simulink model "motoraiHIL"  (R2018b)
settings: Solver=FixedStepDiscrete  StartTime=0.0  StopTime=inf  FixedStep=SAMPLE_TIME  RelTol=1e-3
InitFcn:
  | UserSettings
values from neighbouring files (symbols this model uses):
  ADC_bits = 12    [LQR_control_design.m]    (also in UserSettings.m)
  ADC_Vref = 3.3    [LQR_control_design.m]    (also in UserSettings.m)
  current_gain = 0.5    [LQR_control_design.m]    (also in UserSettings.m)
  current_offset = 1    [LQR_control_design.m]    (also in UserSettings.m)
  DATA_SAMPLING_FREQUENCY = 500    [UserSettings.m]
  ESTIMATION_SAMPLES = 50    [UserSettings.m]
  i_max = 20    [LQG_control_design.m]    (also in LQR_control_design.m; UserSettings.m)
  motorParameters = Parameters()    [UserSettings.m]
  omega_gain = 0.5    [LQR_control_design.m]    (also in UserSettings.m)
  omega_max = 20    [LQG_control_design.m]    (also in LQR_control_design.m; UserSettings.m)
  omega_offset = 1    [LQR_control_design.m]    (also in UserSettings.m)
  PPR = 1000    [LQR_control_design.m]    (also in UserSettings.m)
  SAMPLE_TIME = 5e-5    (= 5e-05)    [UserSettings.m]
  V_ACT = 12    [UserSettings.m]
  v_max = 10    [LQG_control_design.m]    (also in LQR_control_design.m; UserSettings.m)
undefined symbols (not defined in the file or in its folder): myLQR, myREF, parameter_ranges
libraries: neural x230, mbedblockslib x7, dspswit3 x2, dspbuff3 x2, powerlib_meascontrol x2, discretizing x1
(part 1 of 11)
settings Model: ExtModeTrigDuration=10  Creator=Filippo  LastModifiedBy=Filippo
settings OptimizationCC: DefaultParameterBehavior=Inlined  UseDivisionForNetSlopeComputation=on  UseFloatMulNetSlope=on  UseSpecifiedMinMax=on  InlineInvariantSignals=on  EnhancedBackFolding=on  BooleansAsBitfields=on  PassReuseOutputArgsAs=Individual arguments  StateBitsets=on  DataBitsets=on  ZeroExternalMemoryAtStartup=off  ZeroInternalMemoryAtStartup=off  NoFixptDivByZeroProtection=on  EfficientFloat2IntCast=on  LifeSpan=1  MaxStackSize=64  OptimizeBlockOrder=speed  DifferentSizesBufferReuse=on
settings DebuggingCC: SignalInfNanChecking=error  IntegerOverflowMsg=error  ParameterTunabilityLossMsg=error  AssertControl=DisableAll  SFUndirectedBroadcastEventsDiag=error
settings HardwareCC: ProdBitPerPointer=32  ProdBitPerSizeT=32  ProdBitPerPtrDiffT=32  ProdLargestAtomicInteger=Long  ProdLargestAtomicFloat=Double  ProdWordSize=32  ProdLongLongMode=on  ProdHWDeviceType=ARM Compatible->ARM Cortex
settings SFSimCC: CompileTimeRecursionLimit=0  EnableRuntimeRecursion=off  MATLABDynamicMemAlloc=off
settings RTWCC: SystemTargetFile=ert.tlc  HardwareBoard=STM32 Nucleo F411RE  TemplateMakefile=ert_default_tmf  GenerateReport=on  Toolchain=GNU Tools for ARM Embedded Processors  BuildConfiguration=Faster Runs  IncludeHyperlinkInReport=on  LaunchReport=on  GenerateTraceInfo=on  GenerateTraceReport=on  GenerateTraceReportSl=on  GenerateTraceReportSf=on  GenerateTraceReportEml=on  GenerateCodeMetricsReport=on
settings CodeAppCC: ForceParamTrailComments=on  IgnoreCustomStorageClasses=off  OperatorAnnotations=on  SimulinkDataObjDesc=on  SFDataObjDesc=on  CustomSymbolStrGlobalVar=rt$N$M  CustomSymbolStrType=$N$M  CustomSymbolStrFcn=$N$M$F  CustomSymbolStrMacro=$N$M  InsertBlockDesc=on
settings ERTTargetCC: UtilityFuncGeneration=Shared location  IncludeMdlTerminateFcn=off  CombineSignalStateStructs=on  SupportAbsoluteTime=off  SupportComplex=off  SupportNonInlinedSFcns=on  SupportVariableSizeSignals=on  ParenthesesLevel=Maximum  CastingMode=Standards  GenerateSharedConstants=off  InlinedParameterPlacement=NonHierarchical  ERTFilePackagingFormat=CompactWithDataFile  EnableSignedLeftShifts=off  EnableSignedRightShifts=off

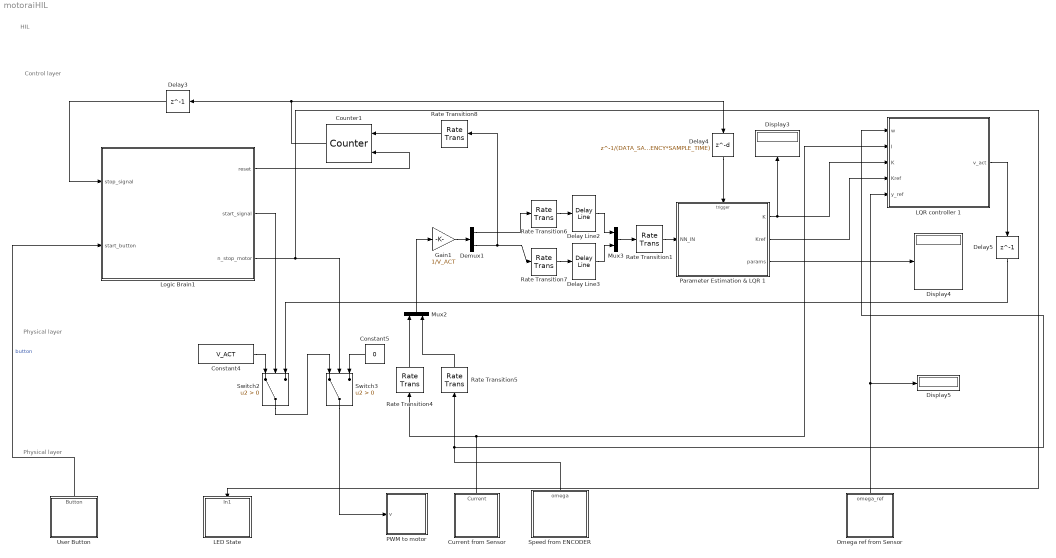
== system motoraiHIL ==
  note: Physical layer
  note: Control layer
  note: HIL
  note: Physical layer
  Constant4 : Constant  Value=V_ACT  SampleTime=SAMPLE_TIME
  Constant5 : Constant  Value=0
  Counter1 : dspswit3/Counter  Direction=Up  CountEvent=Non-zero sample  CounterSize=User defined  MaxCount=(ESTIMATION_SAMPLES)/(DATA_SAMPLING_FREQUENCY*SAMPLE_TIME)  InitialCount=0  Output=Hit  HitValue=(ESTIMATION_SAMPLES)/(DATA_SAMPLING_FREQUENCY*SAMPLE_TIME)  ResetInput=on  SamplesPerFrame=1  Ts=1  CntDtype=double  HitDtype=Logical
  Current from Sensor : Subsystem
      mask Display: image('E:\Università\Magistrale - Advanced Automotive Electronic Engineering\Compliance Design of Automotive Systems\motor-control\MATLAB\images\lowres-INFIN_Icon_Current_02.eps.png');
  Delay Line2 : dspbuff3/Delay Line  siz=50  ic=0  directfeed=off  enable_output=off  hold_output=off  OutputFrames=off
      settings: SourceProductName=DSP System Toolbox  SourceProductBaseCode=DS
  Delay Line3 : dspbuff3/Delay Line  siz=50  ic=0  directfeed=off  enable_output=off  hold_output=off  OutputFrames=off
      settings: SourceProductName=DSP System Toolbox  SourceProductBaseCode=DS
  Delay3 : Delay  DelayLength=1  InitialCondition=0
  Delay4 : Delay  DelayLength=1/(DATA_SAMPLING_FREQUENCY*SAMPLE_TIME)  InitialCondition=0
  Delay5 : Delay  DelayLength=1  InitialCondition=0
  Demux1 : Demux  Outputs=2
  Display3 : Display
  Display4 : Display
  Display5 : Display
  Gain1 : Gain  Gain=1/V_ACT
  LED State : Subsystem
      mask Display: image('E:\Università\Magistrale - Advanced Automotive Electronic Engineering\Compliance Design of Automotive Systems\motor-control\MATLAB\images\led.png');
  LQR controller 1 : Subsystem  TreatAsAtomicUnit=on
  Logic Brain1 : Stateflow chart  TreatAsAtomicUnit=on
  Mux2 : Mux  Inputs=2
  Mux3 : Mux  Inputs=2
  Omega ref from Sensor : Subsystem
      mask Display: image('E:\Università\Magistrale - Advanced Automotive Electronic Engineering\Compliance Design of Automotive Systems\motor-control\MATLAB\images\65193.png');
  PWM to motor : Subsystem
      mask Display: image('E:\Università\Magistrale - Advanced Automotive Electronic Engineering\Compliance Design of Automotive Systems\motor-control\MATLAB\images\PWM-Icon.png');
  Parameter Estimation & LQR 1 : Subsystem  TreatAsAtomicUnit=on
  Rate Transition1 : RateTransition  OutPortSampleTime=SAMPLE_TIME
  Rate Transition{4..7} (4 alike) : RateTransition  OutPortSampleTime=1/DATA_SAMPLING_FREQUENCY
  Rate Transition8 : RateTransition  OutPortSampleTime=SAMPLE_TIME
  Speed from ENCODER : Subsystem
      mask Display: image('E:\Università\Magistrale - Advanced Automotive Electronic Engineering\Compliance Design of Automotive Systems\motor-control\MATLAB\images\Cattura.JPG');
  Switch2 : Switch  Criteria=u2 > Threshold
  Switch3 : Switch  Criteria=u2 > Threshold
  User Button : Subsystem
      mask Display: image('E:\Università\Magistrale - Advanced Automotive Electronic Engineering\Compliance Design of Automotive Systems\motor-control\MATLAB\images\red-start-button-5a28dc2fca5281.8598306415126272478287.jpg');
  wires:
  Rate Transition8/1 -> Counter1/1
  Rate Transition4/1 -> Mux2/1
  Parameter Estimation & LQR 1/1(K) -> Display3/1, LQR controller 1/3(K)
  Speed from ENCODER/1(omega) -> LQR controller 1/1(w), Rate Transition5/1
  Demux1/1 -> Rate Transition6/1
  Counter1/1 -> Delay4/1, Delay3/1
  Parameter Estimation & LQR 1/2(Kref) -> LQR controller 1/4(Kref)
  Current from Sensor/1(Current) -> LQR controller 1/2(I), Rate Transition4/1
  Switch2/1 -> Switch3/1
  Delay Line3/1 -> Mux3/2
  Constant5/1 -> Switch3/3
  Delay Line2/1 -> Mux3/1
  Delay5/1 -> Switch2/3
  User Button/1(Button) -> Logic Brain1/2(start_button)  "button"
  Logic Brain1/2(start_signal) -> Switch2/2
  Constant4/1 -> Switch2/1
  Rate Transition5/1 -> Mux2/2
  Mux2/1 -> Gain1/1
  Delay4/1 -> Parameter Estimation & LQR 1/Trigger
  Mux3/1 -> Rate Transition1/1
  Omega ref from Sensor/1(omega_ref) -> LQR controller 1/5(y_ref), Display5/1
  Switch3/1 -> PWM to motor/1(v)
  Gain1/1 -> Demux1/1
  Rate Transition7/1 -> Delay Line3/1
  Parameter Estimation & LQR 1/3(params) -> Display4/1
  Rate Transition6/1 -> Delay Line2/1
  Logic Brain1/1(reset) -> Counter1/2
  LQR controller 1/1(v_act) -> Delay5/1
  Logic Brain1/3(n_stop_motor) -> LED State/1(In1), Switch3/2
  Demux1/2 -> Rate Transition7/1, Rate Transition8/1
  Delay3/1 -> Logic Brain1/1(stop_signal)
  Rate Transition1/1 -> Parameter Estimation & LQR 1/1(NN_IN)

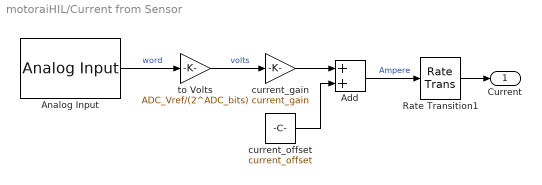
== system motoraiHIL/Current from Sensor ==
  Add : Sum
  Analog Input : mbedblockslib/Analog Input  Pin=PB_0  ReadResultsOnly=off  ConversionTriggerSource=Software  ExternalTriggerType=uint32( 0 )  OutputDataType=double  EnableConversionCompleteNotify=off  EnableOuputStatus=off  SampleTime=1/DATA_SAMPLING_FREQUENCY
      settings: SourceProductName=Simulink Coder Support Package for BBC microbit Board  SourceProductBaseCode=MICROBIT
  Rate Transition1 : RateTransition  OutPortSampleTime=SAMPLE_TIME
  current_gain : Gain  Gain=current_gain
  current_offset : Constant  Value=current_offset  SampleTime=1/DATA_SAMPLING_FREQUENCY
  to Volts : Gain  Gain=ADC_Vref/(2^ADC_bits)
  Current : Outport
  wires:
  Analog Input/1 -> to Volts/1  "word"
  current_gain/1 -> Add/1
  current_offset/1 -> Add/2
  to Volts/1 -> current_gain/1  "volts"
  Add/1 -> Rate Transition1/1  "Ampere"
  Rate Transition1/1 -> Current/1

== system motoraiHIL/LED State ==
  In1 : Inport
  Digital Write : mbedblockslib/Digital Write  Pin=PA_5  Direction=output
      settings: SourceProductName=Simulink Coder Support Package for BBC microbit Board  SourceProductBaseCode=MICROBIT
  NOT : Logic  Operator=NOT  IconShape=distinctive  AllPortsSameDT=off  OutDataTypeStr=boolean
  wires:
  In1/1 -> NOT/1
  NOT/1 -> Digital Write/1

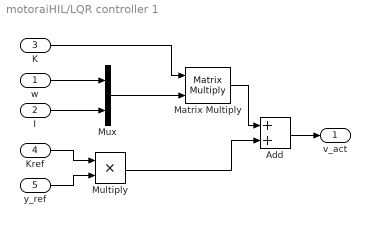
== system motoraiHIL/LQR controller 1 ==
  w : Inport
  I : Inport  Port=2
  K : Inport  Port=3
  Kref : Inport  Port=4
  y_ref : Inport  Port=5
  Add : Sum
  Matrix Multiply : Product  Multiplication=Matrix(*)
  Multiply : Product
  Mux : Mux  Inputs=2
  v_act : Outport
  wires:
  K/1 -> Matrix Multiply/1
  y_ref/1 -> Multiply/2
  Multiply/1 -> Add/2
  Matrix Multiply/1 -> Add/1
  Add/1 -> v_act/1
  I/1 -> Mux/2
  w/1 -> Mux/1
  Kref/1 -> Multiply/1
  Mux/1 -> Matrix Multiply/2

== system motoraiHIL/Omega ref from Sensor ==
  Add : Sum
  Analog Input : mbedblockslib/Analog Input  Pin=PC_0  ReadResultsOnly=off  ConversionTriggerSource=Software  ExternalTriggerType=uint32( 0 )  OutputDataType=double  EnableConversionCompleteNotify=off  EnableOuputStatus=off  SampleTime=-1
      settings: SourceProductName=Simulink Coder Support Package for BBC microbit Board  SourceProductBaseCode=MICROBIT
  omega_gain : Gain  Gain=omega_gain
  omega_offset : Constant  Value=omega_offset
  to Volts : Gain  Gain=ADC_Vref/(2^ADC_bits)
  omega_ref : Outport
  wires:
  Add/1 -> omega_ref/1  "rad/s"
  to Volts/1 -> omega_gain/1  "volts"
  omega_offset/1 -> Add/2
  omega_gain/1 -> Add/1
  Analog Input/1 -> to Volts/1  "word"

== system motoraiHIL/PWM to motor ==
  v : Inport
  Actuation voltage : Constant  Value=V_ACT
  Divide : Product  Inputs=*/
  Divide1 : Product  Inputs=**
  PWM Output : mbedblockslib/PWM Output  Pin=PA_3  EnableInputFrequency=off  InitialFrequency=2000  InitialDutyCycle=50  NotificationType=None
      settings: SourceProductName=Simulink Coder Support Package for BBC microbit Board  SourceProductBaseCode=MICROBIT
  to percentage : Constant  Value=100
  wires:
  Actuation voltage/1 -> Divide/2
  v/1 -> Divide/1
  Divide/1 -> Divide1/1
  to percentage/1 -> Divide1/2
  Divide1/1 -> PWM Output/1

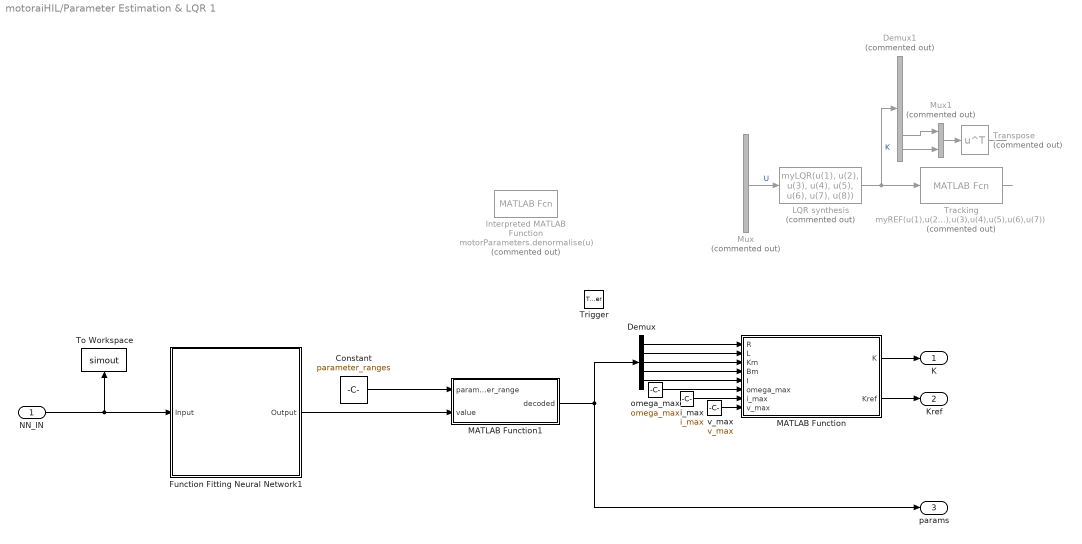
== system motoraiHIL/Parameter Estimation & LQR 1 ==
  NN_IN : Inport
  Trigger : TriggerPort  VariantControl=Variant
  Constant : Constant  Value=parameter_ranges
  Demux : Demux  Outputs=5
  Demux1 : Demux  Commented=on  Outputs=7
  Function Fitting Neural Network1 : Subsystem
      mask help: Function Fitting Neural Network
      mask Display: e = 0.06;c1 = [120 150 230]/255;c2 = ([120 150 230]+0)/383;c3 = ([120 150 230]+128)/383;patch([0 1 1 0],[0 0 1 1],c1);patch([0 1 1 1-e 1-e 0+e],[0 0 1 1-e 0+e 0+e],c2);patch([0 0 1 1-e 0+e 0+e],[0 1 1 1-e 1-e 0+e],c3);plot([0 1 1 0 0],[0 0 1 1 0]);fprintf('NNET');port_label('input',1,' Input');port_label('output',1,'Output ');
  Interpreted MATLAB Function : MATLABFcn  Commented=on  MATLABFcn=motorParameters.denormalise(u)
  LQR synthesis : MATLABFcn  Commented=on  MATLABFcn=myLQR(u(1), u(2), u(3), u(4), u(5), u(6), u(7), u(8))  OutputDimensions=7  Output1D=off
  MATLAB Function : MATLAB Function  TreatAsAtomicUnit=on
  MATLAB Function1 : MATLAB Function  TreatAsAtomicUnit=on
  Mux : Mux  Commented=on  Inputs=8
  Mux1 : Mux  Commented=on  Inputs=2
  To Workspace : ToWorkspace  VariableName=simout  SaveFormat=Timeseries  SampleTime=-1
  Tracking : MATLABFcn  Commented=on  MATLABFcn=myREF(u(1),u(2),u(3),u(4),u(5),u(6),u(7))
  Transpose : Math  Commented=on  Operator=transpose  SaturateOnIntegerOverflow=on
  i_max : Constant  Value=i_max
  omega_max : Constant  Value=omega_max
  v_max : Constant  Value=v_max
  K : Outport
  Kref : Outport  Port=2
  params : Outport  Port=3
  wires:
  Function Fitting Neural Network1/1(Output) -> MATLAB Function1/2(value)
  NN_IN/1 -> Function Fitting Neural Network1/1(Input), To Workspace/1
  MATLAB Function1/1(decoded) -> params/1, Demux/1
  Mux/1 -> LQR synthesis/1  "U"
  i_max/1 -> MATLAB Function/7(i_max)
  omega_max/1 -> MATLAB Function/6(omega_max)
  Demux/5 -> MATLAB Function/5(I)
  Demux/4 -> MATLAB Function/4(Bm)
  Demux/3 -> MATLAB Function/3(Km)
  Demux/2 -> MATLAB Function/2(L)
  Demux/1 -> MATLAB Function/1(R)
  v_max/1 -> MATLAB Function/8(v_max)
  Tracking/1 -> ?
  LQR synthesis/1 -> Demux1/1, Tracking/1  "K"
  Demux1/7 -> Mux1/2
  Demux1/6 -> Mux1/1
  Mux1/1 -> Transpose/1
  Transpose/1 -> ?
  MATLAB Function/1(K) -> K/1
  MATLAB Function/2(Kref) -> Kref/1
  Constant/1 -> MATLAB Function1/1(parameter_range)

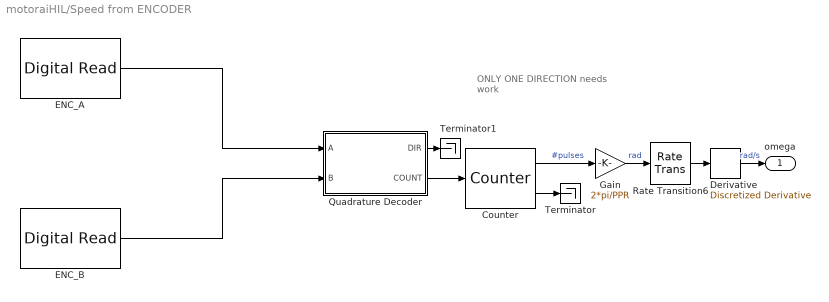
== system motoraiHIL/Speed from ENCODER ==
  note: ONLY ONE DIRECTION
      | needs work
  Counter : dspswit3/Counter  Direction=Up  CountEvent=Rising edge  CounterSize=User defined  MaxCount=255  InitialCount=0  Output=Count and Hit  HitValue=32  ResetInput=off  SamplesPerFrame=1  Ts=1  CntDtype=double  HitDtype=Logical
  Derivative : discretizing/Discretized Derivative  method=tustin  SampleTime=SAMPLE_TIME  Wc=1
  ENC_A : mbedblockslib/Digital Read  Pin=PA_0  Direction=input  SampleTime=1/DATA_SAMPLING_FREQUENCY
      settings: SourceProductName=Simulink Coder Support Package for BBC microbit Board  SourceProductBaseCode=MICROBIT
  ENC_B : mbedblockslib/Digital Read  Pin=PA_1  Direction=input  SampleTime=1/DATA_SAMPLING_FREQUENCY
      settings: SourceProductName=Simulink Coder Support Package for BBC microbit Board  SourceProductBaseCode=MICROBIT
  Gain : Gain  Gain=2*pi/PPR
  Quadrature Decoder : Subsystem
  Rate Transition6 : RateTransition  OutPortSampleTime=SAMPLE_TIME
  Terminator : Terminator
  Terminator1 : Terminator
  omega : Outport
  wires:
  ENC_A/1 -> Quadrature Decoder/1(A)
  ENC_B/1 -> Quadrature Decoder/2(B)
  Quadrature Decoder/2(COUNT) -> Counter/1
  Counter/1 -> Gain/1  "#pulses"
  Gain/1 -> Rate Transition6/1  "rad"
  Derivative/1 -> omega/1  "rad/s"
  Counter/2 -> Terminator/1
  Rate Transition6/1 -> Derivative/1
  Quadrature Decoder/1(DIR) -> Terminator1/1

== system motoraiHIL/User Button ==
  Digital Read : mbedblockslib/Digital Read  Pin=PC_13  Direction=input  SampleTime=-1
      settings: SourceProductName=Simulink Coder Support Package for BBC microbit Board  SourceProductBaseCode=MICROBIT
  Button : Outport
  wires:
  Digital Read/1 -> Button/1

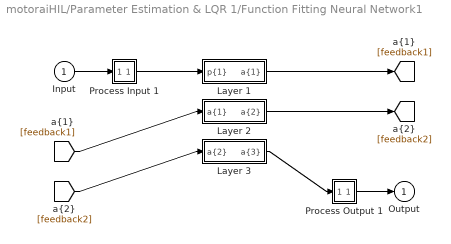
== system motoraiHIL/Parameter Estimation & LQR 1/Function Fitting Neural Network1 ==
  Input : Inport  PortDimensions=100
      mask Display: e = 0.06;c1 = [120 230 180]/255;c2 = ([120 230 180]+0)/(256+128);c3 = ([120 230 180]+128)/(256+128);patch([0 1 1 0],[0 0 1 1],c1);patch([0 1 1 1-e 1-e 0+e],[0 0 1 1-e 0+e 0+e],c2);patch([0 0 1 1-e 0+e 0+e],[0 1 1 1-e 1-e 0+e],c3);plot([0 1 1 0 0],[0 0 1 1 0]);
  Layer 1 : Subsystem
      mask Display: e = 0.06;c1 = [120 150 230]/255;c2 = ([120 150 230]+0)/383;c3 = ([120 150 230]+128)/383;patch([0 1 1 0],[0 0 1 1],c1);patch([0 1 1 1-e 1-e 0+e],[0 0 1 1-e 0+e 0+e],c2);patch([0 0 1 1-e 0+e 0+e],[0 1 1 1-e 1-e 0+e],c3);plot([0 1 1 0 0],[0 0 1 1 0]);
  Layer 2 : Subsystem
      mask Display: e = 0.06;c1 = [120 150 230]/255;c2 = ([120 150 230]+0)/383;c3 = ([120 150 230]+128)/383;patch([0 1 1 0],[0 0 1 1],c1);patch([0 1 1 1-e 1-e 0+e],[0 0 1 1-e 0+e 0+e],c2);patch([0 0 1 1-e 0+e 0+e],[0 1 1 1-e 1-e 0+e],c3);plot([0 1 1 0 0],[0 0 1 1 0]);
  Layer 3 : Subsystem
      mask Display: e = 0.06;c1 = [120 150 230]/255;c2 = ([120 150 230]+0)/383;c3 = ([120 150 230]+128)/383;patch([0 1 1 0],[0 0 1 1],c1);patch([0 1 1 1-e 1-e 0+e],[0 0 1 1-e 0+e 0+e],c2);patch([0 0 1 1-e 0+e 0+e],[0 1 1 1-e 1-e 0+e],c3);plot([0 1 1 0 0],[0 0 1 1 0]);
  Process Input 1 : Subsystem
      mask Display: e = 0.06;c1 = [120 150 230]/255;c2 = ([120 150 230]+0)/383;c3 = ([120 150 230]+128)/383;patch([0 1 1 0],[0 0 1 1],c1);patch([0 1 1 1-e 1-e 0+e],[0 0 1 1-e 0+e 0+e],c2);patch([0 0 1 1-e 0+e 0+e],[0 1 1 1-e 1-e 0+e],c3);plot([0 1 1 0 0],[0 0 1 1 0]);
  Process Output 1 : Subsystem
      mask Display: e = 0.06;c1 = [120 150 230]/255;c2 = ([120 150 230]+0)/383;c3 = ([120 150 230]+128)/383;patch([0 1 1 0],[0 0 1 1],c1);patch([0 1 1 1-e 1-e 0+e],[0 0 1 1-e 0+e 0+e],c2);patch([0 0 1 1-e 0+e 0+e],[0 1 1 1-e 1-e 0+e],c3);plot([0 1 1 0 0],[0 0 1 1 0]);
  Output : Outport  InitialOutput=[0;0;0;0;0]
      mask Display: e = 0.06;c1 = [120 230 180]/255;c2 = ([120 230 180]+0)/(256+128);c3 = ([120 230 180]+128)/(256+128);patch([0 1 1 0],[0 0 1 1],c1);patch([0 1 1 1-e 1-e 0+e],[0 0 1 1-e 0+e 0+e],c2);patch([0 0 1 1-e 0+e 0+e],[0 1 1 1-e 1-e 0+e],c3);plot([0 1 1 0 0],[0 0 1 1 0]);
  wires:
  Input/1 -> Process Input 1/1(x)
  Process Output 1/1(y) -> Output/1
  Process Input 1/1(p) -> Layer 1/1("p{1}")
  Layer 1/1("a{1}") -> [feedback1]
  [feedback1] -> Layer 2/1("a{1} ")
  Layer 2/1("a{2}") -> [feedback2]
  [feedback2] -> Layer 3/1("a{2} ")
  Layer 3/1("a{3}") -> Process Output 1/1(a)

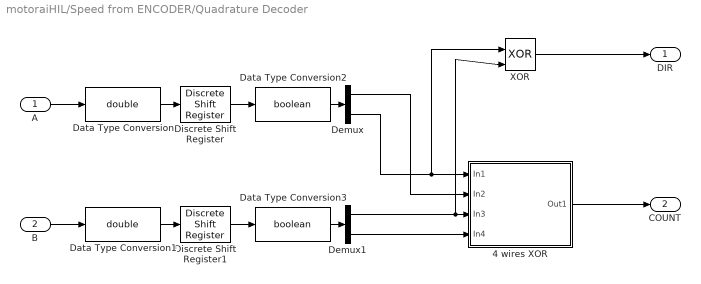
== system motoraiHIL/Speed from ENCODER/Quadrature Decoder ==
  A : Inport
  B : Inport  Port=2
  4 wires XOR : Subsystem
  Data Type Conversion : DataTypeConversion  OutDataTypeStr=double
  Data Type Conversion1 : DataTypeConversion  OutDataTypeStr=double
  Data Type Conversion2 : DataTypeConversion  OutDataTypeStr=boolean
  Data Type Conversion3 : DataTypeConversion  OutDataTypeStr=boolean
  Demux : Demux  Outputs=2
  Demux1 : Demux  Outputs=2
  Discrete Shift Register : powerlib_meascontrol/Additional Components/Discrete Shift Register  NSamples=2  InitialValue=0  Ts=1/DATA_SAMPLING_FREQUENCY
      settings: SourceProductName=Simscape Electrical  SourceProductBaseCode=PS
  Discrete Shift Register1 : powerlib_meascontrol/Additional Components/Discrete Shift Register  NSamples=2  InitialValue=0  Ts=1/DATA_SAMPLING_FREQUENCY
      settings: SourceProductName=Simscape Electrical  SourceProductBaseCode=PS
  XOR : Logic  Operator=XOR  IconShape=distinctive  AllPortsSameDT=off  OutDataTypeStr=boolean
  DIR : Outport
  COUNT : Outport  Port=2
  wires:
  4 wires XOR/1(Out1) -> COUNT/1
  Demux/1 -> 4 wires XOR/2(In2)
  Demux/2 -> XOR/1, 4 wires XOR/1(In1)
  Demux1/1 -> XOR/2, 4 wires XOR/3(In3)
  Demux1/2 -> 4 wires XOR/4(In4)
  XOR/1 -> DIR/1
  A/1 -> Data Type Conversion/1
  Data Type Conversion/1 -> Discrete Shift Register/1
  Data Type Conversion1/1 -> Discrete Shift Register1/1
  B/1 -> Data Type Conversion1/1
  Discrete Shift Register/1 -> Data Type Conversion2/1
  Data Type Conversion2/1 -> Demux/1
  Discrete Shift Register1/1 -> Data Type Conversion3/1
  Data Type Conversion3/1 -> Demux1/1

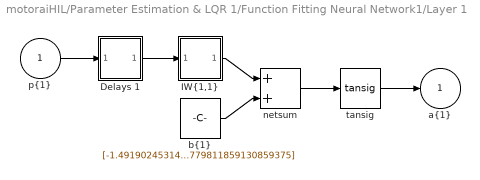
== system motoraiHIL/Parameter Estimation & LQR 1/Function Fitting Neural Network1/Layer 1 ==
  "p{1}" : Inport  PortDimensions=100
      mask Display: e = 0.06;c1 = [120 230 180]/255;c2 = ([120 230 180]+0)/(256+128);c3 = ([120 230 180]+128)/(256+128);patch([0 1 1 0],[0 0 1 1],c1);patch([0 1 1 1-e 1-e 0+e],[0 0 1 1-e 0+e 0+e],c2);patch([0 0 1 1-e 0+e 0+e],[0 1 1 1-e 1-e 0+e],c3);plot([0 1 1 0 0],[0 0 1 1 0]);
  Delays 1 : Subsystem
      mask Display: e = 0.06;c1 = [120 150 230]/255;c2 = ([120 150 230]+0)/383;c3 = ([120 150 230]+128)/383;patch([0 1 1 0],[0 0 1 1],c1);patch([0 1 1 1-e 1-e 0+e],[0 0 1 1-e 0+e 0+e],c2);patch([0 0 1 1-e 0+e 0+e],[0 1 1 1-e 1-e 0+e],c3);plot([0 1 1 0 0],[0 0 1 1 0]);disp('0');
  "IW{1,1}" : Subsystem
      mask Display: e = 0.06;c1 = [120 150 230]/255;c2 = ([120 150 230]+0)/383;c3 = ([120 150 230]+128)/383;patch([0 1 1 0],[0 0 1 1],c1);patch([0 1 1 1-e 1-e 0+e],[0 0 1 1-e 0+e 0+e],c2);patch([0 0 1 1-e 0+e 0+e],[0 1 1 1-e 1-e 0+e],c3);plot([0 1 1 0 0],[0 0 1 1 0]);disp('W');
  "b{1}" : Constant  Value=[-1.4919024531456328563905344708473421633243560791015625;-3.324035791624780689090812302310951054096221923828125;-4.13456829414457160964957438409328460693359375;-1.836723010850963788698209100402891635894775390625;-1.4091586472986861178213757739285938441753387451171875;4.970534426222030788267147727310657501220703125;-1.43306901188916668843376100994646549224853515625;2.2279527488562589354614829062484204769134521484375;1.328259519520753162424853144329972565174102783203125;-2.020758521084016212654432820272631943225860595703125;2.16421482148424981772905084653757512569427490234375;4.20171892986421458004997475654818117618560791015625;-1.274483640968156805683975107967853546142578125;3.60720938587216988224781744065694510936737060546875;1.292942336452524099144056890509091317653656005859375;-3.5397007250318797133559201029129326343536376953125;-1.786737363460142891113946461700834333896636962890625;1.213072407322157264530915199429728090763092041015625;1.9368639177277608975913381073041819036006927490234375;-1.183644809824522692309756166650913655757904052734375;2.73605642718861030715515880729071795940399169921875;1.1750795504756628151454833641764707863330841064453125;3.63292805917073824417684591026045382022857666015625;-1.92529254928110304945221287198364734649658203125;1.1217023889151123139384935711859725415706634521484375;-2.19969076054615708670780804823152720928192138671875;2.46465318930706001054886655765585601329803466796875;3.519379580867114665210237944847904145717620849609375;-3.510986477319951060138691900647245347499847412109375;-3.362066143879420376805455816793255507946014404296875;-3.2372647299874319770651709404774010181427001953125;3.03867276328607172075635389774106442928314208984375;-0.95029259580614944269427724066190421581268310546875;-0.92459214678282986010771082874271087348461151123046875;-3.124414120087879442877465407946147024631500244140625;-0.9353827043479390201952128336415626108646392822265625;2.254725896910846127951799644506536424160003662109375;-0.834472845713261524025483595323748886585235595703125;0.8913529491038101326694231829605996608734130859375;1.8812399288297274591030827650683932006359100341796875;1.8531337308741366864950350645813159644603729248046875;-0.78517889590191647375405636921641416847705841064453125;-2.071393544628578720079303820966742932796478271484375;-0.72892888199155081441205084047396667301654815673828125;-2.036226452743351789109738092520274221897125244140625;-1.773124276466413906661045984947122633457183837890625;-2.2121414640265779638639287441037595272064208984375;-1.778784910497580806776340978103689849376678466796875;0.705785377512704759084272154723294079303741455078125;1.43067917044885462019010446965694427490234375;1.9257026622676374216780459391884505748748779296875;1.203076947037368338300211689784191548824310302734375;-1.893163059372398482338439862360246479511260986328125;-1.179426651812485626891202628030441701412200927734375;-1.7137817964897175126992578952922485768795013427734375;0.50012141067598558930029639668646268546581268310546875;0.50729081569372258542216513887979090213775634765625;-0.5292961890166030247684147980180568993091583251953125;-1.3484296254140968329693350824527442455291748046875;0.513737331515440320828247422468848526477813720703125;1.1396321098108075364763180914451368153095245361328125;-0.70346486670542685004647864843718707561492919921875;-1.98838173638628479267254078877158463001251220703125;-0.8396818628790925220783947224845178425312042236328125;0.27107396715911846740709734149277210235595703125;-0.537527917836701618625738774426281452178955078125;-0.6952060242946085377724330101045779883861541748046875;-0.7886526911267870421085035559372045099735260009765625;1.17531905111180723366715028532780706882476806640625;0.290825141576465273640650366360205225646495819091796875;0.1480170973065546846658691038101096637547016143798828125;0.2100331078052113109588816541872802190482616424560546875;0.4979086865674993145347571044112555682659149169921875 ...(+5122 chars)]
      mask Display: e = 0.06;c1 = [120 150 230]/255;c2 = ([120 150 230]+0)/383;c3 = ([120 150 230]+128)/383;patch([0 1 1 0],[0 0 1 1],c1);patch([0 1 1 1-e 1-e 0+e],[0 0 1 1-e 0+e 0+e],c2);patch([0 0 1 1-e 0+e 0+e],[0 1 1 1-e 1-e 0+e],c3);plot([0 1 1 0 0],[0 0 1 1 0]);disp('b');
  netsum : Sum  Inputs=2  SaturateOnIntegerOverflow=on  InputSameDT=on  OutDataTypeStr=Inherit: Same as first input
      mask Display: e = 0.06;c1 = [120 150 230]/255;c2 = ([120 150 230]+0)/383;c3 = ([120 150 230]+128)/383;patch([0 1 1 0],[0 0 1 1],c1);patch([0 1 1 1-e 1-e 0+e],[0 0 1 1-e 0+e 0+e],c2);patch([0 0 1 1-e 0+e 0+e],[0 1 1 1-e 1-e 0+e],c3);plot([0 1 1 0 0],[0 0 1 1 0]);disp('+');
  tansig : neural/Transfer Functions/tansig
  "a{1}" : Outport  InitialOutput=[0;0;0;0;0;0;0;0;0;0;0;0;0;0;0;0;0;0;0;0;0;0;0;0;0;0;0;0;0;0;0;0;0;0;0;0;0;0;0;0;0;0;0;0;0;0;0;0;0;0;0;0;0;0;0;0;0;0;0;0;0;0;0;0;0;0;0;0;0;0;0;0;0;0;0;0;0;0;0;0;0;0;0;0;0;0;0;0;0;0;0;0;0;0;0;0;0;0;0;0;0;0;0;0;0;0;0;0;0;0;0;0;0;0;0;0;0;0;0;0;0;0;0;0;0;0;0;0;0;0;0;0;0;0;0;0;0;0;0;0;0;0;0;0;0;0;0;0;0;0;0;0;0;0;0;0;0;0;0;0;0;0;0;0;0;0]
      mask Display: e = 0.06;c1 = [120 230 180]/255;c2 = ([120 230 180]+0)/(256+128);c3 = ([120 230 180]+128)/(256+128);patch([0 1 1 0],[0 0 1 1],c1);patch([0 1 1 1-e 1-e 0+e],[0 0 1 1-e 0+e 0+e],c2);patch([0 0 1 1-e 0+e 0+e],[0 1 1 1-e 1-e 0+e],c3);plot([0 1 1 0 0],[0 0 1 1 0]);
  wires:
  "p{1}"/1 -> Delays 1/1("p{1}")
  Delays 1/1("pd{1,1}") -> "IW{1,1}"/1("pd{1,1}")
  "IW{1,1}"/1("iz{1,1}") -> netsum/1
  "b{1}"/1 -> netsum/2
  netsum/1 -> tansig/1
  tansig/1 -> "a{1}"/1

== system motoraiHIL/Parameter Estimation & LQR 1/Function Fitting Neural Network1/Layer 2 ==
  "a{1} " : Inport  PortDimensions=166
      mask Display: e = 0.06;c1 = [120 230 180]/255;c2 = ([120 230 180]+0)/(256+128);c3 = ([120 230 180]+128)/(256+128);patch([0 1 1 0],[0 0 1 1],c1);patch([0 1 1 1-e 1-e 0+e],[0 0 1 1-e 0+e 0+e],c2);patch([0 0 1 1-e 0+e 0+e],[0 1 1 1-e 1-e 0+e],c3);plot([0 1 1 0 0],[0 0 1 1 0]);
  Delays 1 : Subsystem
      mask Display: e = 0.06;c1 = [120 150 230]/255;c2 = ([120 150 230]+0)/383;c3 = ([120 150 230]+128)/383;patch([0 1 1 0],[0 0 1 1],c1);patch([0 1 1 1-e 1-e 0+e],[0 0 1 1-e 0+e 0+e],c2);patch([0 0 1 1-e 0+e 0+e],[0 1 1 1-e 1-e 0+e],c3);plot([0 1 1 0 0],[0 0 1 1 0]);disp('0');
  "LW{2,1}" : Subsystem
      mask Display: e = 0.06;c1 = [120 150 230]/255;c2 = ([120 150 230]+0)/383;c3 = ([120 150 230]+128)/383;patch([0 1 1 0],[0 0 1 1],c1);patch([0 1 1 1-e 1-e 0+e],[0 0 1 1-e 0+e 0+e],c2);patch([0 0 1 1-e 0+e 0+e],[0 1 1 1-e 1-e 0+e],c3);plot([0 1 1 0 0],[0 0 1 1 0]);disp('W');
  "b{2}" : Constant  Value=[-1.520928303378276336133012591744773089885711669921875;-1.442345723903466936377526508294977247714996337890625;1.3487681572279870412245372790494002401828765869140625;1.2900091814729908179515405208803713321685791015625;1.254657124683530522446517352364026010036468505859375;0.9151432308450202501859394033090211451053619384765625;1.1279606934451014144116243187454529106616973876953125;-1.1154275576791727875303195105516351759433746337890625;0.9503957846484436533529560620081610977649688720703125;1.03561980993273028417434034054167568683624267578125;-0.8830656987881109198923468284192495048046112060546875;-0.82221109593234142920437079737894237041473388671875;-0.72784097080261556111935306034865789115428924560546875;0.72939735869099597831421988303191028535366058349609375;-0.67942659210886813259122618546825833618640899658203125;0.622891161288141592677902735886164009571075439453125;0.63674542139648881988733819525805301964282989501953125;-0.52233615361827145928685922626755200326442718505859375;0.5713068549425848186018583874101750552654266357421875;0.3908775031863902515993913766578771173954010009765625;-0.360205945107947289596239670572686009109020233154296875;-0.18364190528169610505671016653650440275669097900390625;0.240861819890472117489110814858577214181423187255859375;-0.324442685216406123682730822110897861421108245849609375;0.136431819003711207738405164491268806159496307373046875;-0.021882514272934895649402875505984411574900150299072265625;-0.07776102887128853724529875535154133103787899017333984375;0.055173943234047499728500696392075042240321636199951171875;-0.1698227426799343298124966850082273595035076141357421875;0.18841882424478983981686042170622386038303375244140625;-0.1292456631537711453372452297116979025304317474365234375;0.26032811162127067472482622179086320102214813232421875;0.220157600554504673251443591652787290513515472412109375;0.3740273551414781127988362641190178692340850830078125;-0.43518440826602311499726738475146703422069549560546875;0.454202361424174527737562812035321258008480072021484375;0.3994401859903178308996984924306161701679229736328125;-0.6009069267007591808038569070049561560153961181640625;0.77440017118956394615025828898069448769092559814453125;-0.72802761451480879628661568858660757541656494140625;-0.64036651201171945757550929556600749492645263671875;-0.67856384971911498649177474362659268081188201904296875;0.86886064903449611307451050379313528537750244140625;-0.836084653311689240950954626896418631076812744140625;-0.97369603472221688544863127390271984040737152099609375;-1.023860528231684607902707284665666520595550537109375;0.9621481931948225874151603420614264905452728271484375;1.1401462963482951185056890608393587172031402587890625;-1.0581323818203356434963779975078068673610687255859375;1.276565058012384401564531799522228538990020751953125;1.2876287672258384109369444558979012072086334228515625;-1.3856148738555369437364106488530524075031280517578125;1.405228042441858615774208374205045402050018310546875;1.49501934411344716835401413845829665660858154296875]
      mask Display: e = 0.06;c1 = [120 150 230]/255;c2 = ([120 150 230]+0)/383;c3 = ([120 150 230]+128)/383;patch([0 1 1 0],[0 0 1 1],c1);patch([0 1 1 1-e 1-e 0+e],[0 0 1 1-e 0+e 0+e],c2);patch([0 0 1 1-e 0+e 0+e],[0 1 1 1-e 1-e 0+e],c3);plot([0 1 1 0 0],[0 0 1 1 0]);disp('b');
  netsum : Sum  Inputs=2  SaturateOnIntegerOverflow=on  InputSameDT=on  OutDataTypeStr=Inherit: Same as first input
      mask Display: e = 0.06;c1 = [120 150 230]/255;c2 = ([120 150 230]+0)/383;c3 = ([120 150 230]+128)/383;patch([0 1 1 0],[0 0 1 1],c1);patch([0 1 1 1-e 1-e 0+e],[0 0 1 1-e 0+e 0+e],c2);patch([0 0 1 1-e 0+e 0+e],[0 1 1 1-e 1-e 0+e],c3);plot([0 1 1 0 0],[0 0 1 1 0]);disp('+');
  tansig : neural/Transfer Functions/tansig
  "a{2}" : Outport  InitialOutput=[0;0;0;0;0;0;0;0;0;0;0;0;0;0;0;0;0;0;0;0;0;0;0;0;0;0;0;0;0;0;0;0;0;0;0;0;0;0;0;0;0;0;0;0;0;0;0;0;0;0;0;0;0;0]
      mask Display: e = 0.06;c1 = [120 230 180]/255;c2 = ([120 230 180]+0)/(256+128);c3 = ([120 230 180]+128)/(256+128);patch([0 1 1 0],[0 0 1 1],c1);patch([0 1 1 1-e 1-e 0+e],[0 0 1 1-e 0+e 0+e],c2);patch([0 0 1 1-e 0+e 0+e],[0 1 1 1-e 1-e 0+e],c3);plot([0 1 1 0 0],[0 0 1 1 0]);
  wires:
  "a{1} "/1 -> Delays 1/1("p{2}")
  Delays 1/1("pd{2,1}") -> "LW{2,1}"/1("ad{2,1}")
  "LW{2,1}"/1("lz{2,1}") -> netsum/1
  "b{2}"/1 -> netsum/2
  netsum/1 -> tansig/1
  tansig/1 -> "a{2}"/1

== system motoraiHIL/Parameter Estimation & LQR 1/Function Fitting Neural Network1/Layer 3 ==
  "a{2} " : Inport  PortDimensions=54
      mask Display: e = 0.06;c1 = [120 230 180]/255;c2 = ([120 230 180]+0)/(256+128);c3 = ([120 230 180]+128)/(256+128);patch([0 1 1 0],[0 0 1 1],c1);patch([0 1 1 1-e 1-e 0+e],[0 0 1 1-e 0+e 0+e],c2);patch([0 0 1 1-e 0+e 0+e],[0 1 1 1-e 1-e 0+e],c3);plot([0 1 1 0 0],[0 0 1 1 0]);
  Delays 1 : Subsystem
      mask Display: e = 0.06;c1 = [120 150 230]/255;c2 = ([120 150 230]+0)/383;c3 = ([120 150 230]+128)/383;patch([0 1 1 0],[0 0 1 1],c1);patch([0 1 1 1-e 1-e 0+e],[0 0 1 1-e 0+e 0+e],c2);patch([0 0 1 1-e 0+e 0+e],[0 1 1 1-e 1-e 0+e],c3);plot([0 1 1 0 0],[0 0 1 1 0]);disp('0');
  "LW{3,2}" : Subsystem
      mask Display: e = 0.06;c1 = [120 150 230]/255;c2 = ([120 150 230]+0)/383;c3 = ([120 150 230]+128)/383;patch([0 1 1 0],[0 0 1 1],c1);patch([0 1 1 1-e 1-e 0+e],[0 0 1 1-e 0+e 0+e],c2);patch([0 0 1 1-e 0+e 0+e],[0 1 1 1-e 1-e 0+e],c3);plot([0 1 1 0 0],[0 0 1 1 0]);disp('W');
  "b{3}" : Constant  Value=[-0.87239417235159566477165071773924864828586578369140625;-0.104613818761169319326853610618854872882366180419921875;-0.5139553195383417261155045707710087299346923828125;-0.848982359275880948956682914285920560359954833984375;0.251747456969745819765904570886050350964069366455078125]
      mask Display: e = 0.06;c1 = [120 150 230]/255;c2 = ([120 150 230]+0)/383;c3 = ([120 150 230]+128)/383;patch([0 1 1 0],[0 0 1 1],c1);patch([0 1 1 1-e 1-e 0+e],[0 0 1 1-e 0+e 0+e],c2);patch([0 0 1 1-e 0+e 0+e],[0 1 1 1-e 1-e 0+e],c3);plot([0 1 1 0 0],[0 0 1 1 0]);disp('b');
  netsum : Sum  Inputs=2  SaturateOnIntegerOverflow=on  InputSameDT=on  OutDataTypeStr=Inherit: Same as first input
      mask Display: e = 0.06;c1 = [120 150 230]/255;c2 = ([120 150 230]+0)/383;c3 = ([120 150 230]+128)/383;patch([0 1 1 0],[0 0 1 1],c1);patch([0 1 1 1-e 1-e 0+e],[0 0 1 1-e 0+e 0+e],c2);patch([0 0 1 1-e 0+e 0+e],[0 1 1 1-e 1-e 0+e],c3);plot([0 1 1 0 0],[0 0 1 1 0]);disp('+');
  purelin : neural/Transfer Functions/purelin
  "a{3}" : Outport  InitialOutput=[0;0;0;0;0]
      mask Display: e = 0.06;c1 = [120 230 180]/255;c2 = ([120 230 180]+0)/(256+128);c3 = ([120 230 180]+128)/(256+128);patch([0 1 1 0],[0 0 1 1],c1);patch([0 1 1 1-e 1-e 0+e],[0 0 1 1-e 0+e 0+e],c2);patch([0 0 1 1-e 0+e 0+e],[0 1 1 1-e 1-e 0+e],c3);plot([0 1 1 0 0],[0 0 1 1 0]);
  wires:
  "a{2} "/1 -> Delays 1/1("p{3}")
  Delays 1/1("pd{3,2}") -> "LW{3,2}"/1("ad{3,2}")
  "LW{3,2}"/1("lz{3,2}") -> netsum/1
  "b{3}"/1 -> netsum/2
  netsum/1 -> purelin/1
  purelin/1 -> "a{3}"/1

== system motoraiHIL/Parameter Estimation & LQR 1/Function Fitting Neural Network1/Process Input 1 ==
  x : Inport  PortDimensions=100
      mask Display: e = 0.06;c1 = [120 230 180]/255;c2 = ([120 230 180]+0)/(256+128);c3 = ([120 230 180]+128)/(256+128);patch([0 1 1 0],[0 0 1 1],c1);patch([0 1 1 1-e 1-e 0+e],[0 0 1 1-e 0+e 0+e],c2);patch([0 0 1 1-e 0+e 0+e],[0 1 1 1-e 1-e 0+e],c3);plot([0 1 1 0 0],[0 0 1 1 0]);
  mapminmax : neural/Processing Functions/mapminmax  xmin=[-1;-1.26350567994937601490335055132;-1.45779194171306336613724852214;-1.36794318155885452625852849451;-1.40652059057718648027446306514;-1.43958045883019525312818132079;-1.34967731497964393838628893718;-1.42650496628851963798467750166;-1.44264268962705100030063931627;-1.32567644404435158733690514055;-1.32759927049568804413581801782;-1.33860446697644430713580732117;-1.35959778550194831936437367403;-1.40971952026102376187566278531;-1.42393990562562655632916630566;-1.35407695415979101305481435702;-1.34127328184212313288981022197;-1.4142183382155704141069918478;-1.44144327279884221226780027791;-1.45025775586362448699162541743;-1.37108564425775880657454308675;-1.2752655773992116472470570443;-1.34437010368871412424596201163;-1.35283668647277055541167101183;-1.41490946112968996040137881209;-1.4273478559274812571544543971;-1.39153152433639948348798043298;-1.39864298461023239816825025628;-1.46429097798899721105669868848;-1.49107518875616662512584298383;-1.529083044953432057866393734;-1.54862613192399622974448902823;-1.53390533988444666135819716146;-1.48736069695304640170263610344;-1.4119570693901180025164876497;-1.31108856905252268987283059687;-1.29037317340084989325532660587;-1.26871431613284801898089426686;-1.22683127725529383944547134888;-1.19957497820095282392571789387;-1.19409006469055190002848121367;-1.22010821118502943427586160396;-1.27241327402137471835885662585;-1.30997428004248495092554094299;-1.3328643122674359577928271392;-1.38915011871117122232988094765;-1.43399344956055574407116637303;-1.46389693278115395891347816359;-1.47938813761115217637609475787;-1.48109303160397121068569958879;-1;0.000316686467929807853680795881601;0.000636034201779292441766844312667;0.000954603056429548799469153586017;0.00127316755314685206915137349881;0.00159172769199081754094848850656;0.00191028347302105963763374507636;0.00222883489629719213145908618401;0.00254738196187882749363384782271;0.00286592466982557884588866947695;0.00318446302019705605734767317472;0.0035029970130528707318584569208;0.00382152664845263100382166676638;0.00414005192645594717604229373364;0.00445857284712242608187837689115;0.00477708941051167585573056229009;0.00509560161668330246359515101062;0.00541410946569691013674496815611;0.00573261295761210484117631480672;0.00605111209248849080816201606581;0.00636960687038566966688968307153;0.00668809729136324564863214092725;0.0070065833554808186478535247943;0.00732506506279799029374144581084;0.0076435424133743604807600391382;0.00796201540726952650128822597253;0.00828048404454308911715187946356;0.00859894832525464301864470684222;0.00891740824946378636550736729305;0.00923586381723011558275704402377;0.00955431502861322362596396828849;0.00987276188367270692014532329495;0.0101912043824681566861478643204;0.0105096425250591658795418226191;0.0108280763115053257211739534682;0.0111465057418662309013379640987;0.0114649308162014657019867058807;0.0117833515345706230786904100682;0.0121017678970332890481254040083;0.0124201799036490530964149670012;0.0127385875544774995055119504173;0.0130569908495782177615396335568;0.0133753897890107938811743437668;0.0136937843728348052074750285101;0.0140121746011098412265649670871;0.0143305604738954827509500589144;0.0146489419912513123278596793853;0.0149673191532369125045232038929;0.0152856919599118571545526279465;0.0156040604113357340293477548698]  xmax=[1;9.77558261162738517668913118541;9.75881586242053344903979450464;9.78864168413107726962607557653;9.79298419894775307170675660018;9.81366015826116111497867677826;9.85534479834922549912334943656;9.86154371845024257936529465951;9.85375948660742473350637737894;9.84051249845274256244920252357;9.82517860083801863879671145696;9.80909497209382408300371025689;9.79279091499302012380212545395;9.77647559327876969348380953306;9.76023131103977448219666257501;9.74409010510114015346516680438;9.72806409689381013095044181682;9.71215752020834166557960998034;9.70362022607610974489489308326;9.69717634491477653568836103659;9.69073678123346660129300289555;9.6843015321394183558822987834;9.67787059474180111351415689569;9.67144396615172752262878930196;9.66502164348224468426451494452;9.65860362384832527027356263716;9.6521899043668923923178226687;9.64578048215678407473205879796;9.63937535433877634716282045702;9.63297451803557613914108515019;9.62657797037181239829806145281;9.62018570847404497214938601246;9.61379772947075572631092654774;9.60741403049235742628297884949;9.60103460867117597388187277829;9.59465946114146461809468746651;9.58828858503939507329505431699;9.58192197750305574288631760282;9.57555963567246060108573146863;9.5692015566895278766423871275;9.56284773769810136911928566406;9.55649817584393268532494403189;9.55015286827468656838391325437;9.54381181213994089773677842459;9.53747500459117958371280110441;9.53114244278179789660043752519;9.52481412386710069029049918754;9.51849004500429707320563466055;9.51217020335249152651613258058;9.50585459607271054949251265498;1;711.036620845298557469504885375;908.09461829969984592025866732;1065.74551307727915627765469253;1154.74341552607484118198044598;1062.81126672770596996997483075;1170.50358266186276523512788117;1182.28868770958638378942850977;1116.58008730226833904453087598;1105.97266991650781164935324341;1214.18363308344737561128567904;1290.00729100976445806736592203;1330.16688837542392320756334811;1333.69883813070896394492592663;1301.91506230633126506290864199;1308.45224645158737075689714402;1297.87291420175779421697370708;1270.51252622542983772291336209;1229.24939721375403678393922746;1177.2948015568138089292915538;1118.01724187482614070177078247;1058.56420762211905639560427517;1044.65477641202505765249952674;1029.64231779294300395122263581;1063.6730122679089163284515962;1094.31361039283137870370410383;1120.47353422336914263723883778;1142.07393835220773326000198722;1159.08624747300586932396981865;1171.53031476077148909098468721;1179.47216013110983112710528076;1183.02132950156828883336856961;1182.32791833138230686017777771;1177.57930433214505683281458914;1168.99663532754334482888225466;1156.83111880663022930093575269;1141.36015977841339008591603488;1122.88339311652725882595404983;1101.71865570623822350171394646;1080.90359756934344659384805709;1052.66338808843147489824332297;1025.46331611498521851899567991;996.948390895620036644686479121;976.696589730229561610030941665;982.262695894934608986659441143;983.478844881539544076076708734;980.72180310446753992437152192;974.933604436009204619040247053;974.933604436009204619040247053;974.933604436009204619040247053]  ymin=-1  ymax=1
  p : Outport  PortDimensions=100
      mask Display: e = 0.06;c1 = [120 230 180]/255;c2 = ([120 230 180]+0)/(256+128);c3 = ([120 230 180]+128)/(256+128);patch([0 1 1 0],[0 0 1 1],c1);patch([0 1 1 1-e 1-e 0+e],[0 0 1 1-e 0+e 0+e],c2);patch([0 0 1 1-e 0+e 0+e],[0 1 1 1-e 1-e 0+e],c3);plot([0 1 1 0 0],[0 0 1 1 0]);
  wires:
  x/1 -> mapminmax/1
  mapminmax/1 -> p/1

== system motoraiHIL/Parameter Estimation & LQR 1/Function Fitting Neural Network1/Process Output 1 ==
  a : Inport  PortDimensions=5
      mask Display: e = 0.06;c1 = [120 230 180]/255;c2 = ([120 230 180]+0)/(256+128);c3 = ([120 230 180]+128)/(256+128);patch([0 1 1 0],[0 0 1 1],c1);patch([0 1 1 1-e 1-e 0+e],[0 0 1 1-e 0+e 0+e],c2);patch([0 0 1 1-e 0+e 0+e],[0 1 1 1-e 1-e 0+e],c3);plot([0 1 1 0 0],[0 0 1 1 0]);
  mapminmax_reverse : neural/Processing Functions/mapminmax_reverse  xmin=[5.01960631904552201376645825803e-06;1.95643928717625925628453842364e-05;8.06619515891782157268607988954e-06;6.33421461537775343231260194443e-06;1.95008388282902345167713065166e-05]  xmax=[0.999951993155747786978793101298;0.999943110312290106556076807465;0.999873910389593500980254248134;0.999966563960045240477825245762;0.999899782730856667711805130239]  ymin=-1  ymax=1
  y : Outport  PortDimensions=5
      mask Display: e = 0.06;c1 = [120 230 180]/255;c2 = ([120 230 180]+0)/(256+128);c3 = ([120 230 180]+128)/(256+128);patch([0 1 1 0],[0 0 1 1],c1);patch([0 1 1 1-e 1-e 0+e],[0 0 1 1-e 0+e 0+e],c2);patch([0 0 1 1-e 0+e 0+e],[0 1 1 1-e 1-e 0+e],c3);plot([0 1 1 0 0],[0 0 1 1 0]);
  wires:
  a/1 -> mapminmax_reverse/1
  mapminmax_reverse/1 -> y/1

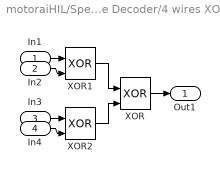
== system motoraiHIL/Speed from ENCODER/Quadrature Decoder/4 wires XOR ==
  In1 : Inport
  In2 : Inport  Port=2
  In3 : Inport  Port=3
  In4 : Inport  Port=4
  XOR : Logic  Operator=XOR  IconShape=distinctive  AllPortsSameDT=off  OutDataTypeStr=boolean
  XOR1 : Logic  Operator=XOR  IconShape=distinctive  AllPortsSameDT=off  OutDataTypeStr=boolean
  XOR2 : Logic  Operator=XOR  IconShape=distinctive  AllPortsSameDT=off  OutDataTypeStr=boolean
  Out1 : Outport
  wires:
  In1/1 -> XOR1/1
  XOR2/1 -> XOR/2
  XOR1/1 -> XOR/1
  XOR/1 -> Out1/1
  In3/1 -> XOR2/1
  In2/1 -> XOR1/2
  In4/1 -> XOR2/2

== system motoraiHIL/Parameter Estimation & LQR 1/Function Fitting Neural Network1/Layer 1/Delays 1 ==
  "p{1}" : Inport  PortDimensions=100
      mask Display: e = 0.06;c1 = [120 230 180]/255;c2 = ([120 230 180]+0)/(256+128);c3 = ([120 230 180]+128)/(256+128);patch([0 1 1 0],[0 0 1 1],c1);patch([0 1 1 1-e 1-e 0+e],[0 0 1 1-e 0+e 0+e],c2);patch([0 0 1 1-e 0+e 0+e],[0 1 1 1-e 1-e 0+e],c3);plot([0 1 1 0 0],[0 0 1 1 0]);
  mux : Mux  Inputs=1
      mask Display: e = 0.06;c1 = [120 150 230]/255;c2 = ([120 150 230]+0)/383;c3 = ([120 150 230]+128)/383;patch([0 1 1 0],[0 0 1 1],c1);patch([0 1 1 1-e 1-e 0+e],[0 0 1 1-e 0+e 0+e],c2);patch([0 0 1 1-e 0+e 0+e],[0 1 1 1-e 1-e 0+e],c3);plot([0 1 1 0 0],[0 0 1 1 0]);disp('Mux')
  "pd{1,1}" : Outport
      mask Display: e = 0.06;c1 = [120 230 180]/255;c2 = ([120 230 180]+0)/(256+128);c3 = ([120 230 180]+128)/(256+128);patch([0 1 1 0],[0 0 1 1],c1);patch([0 1 1 1-e 1-e 0+e],[0 0 1 1-e 0+e 0+e],c2);patch([0 0 1 1-e 0+e 0+e],[0 1 1 1-e 1-e 0+e],c3);plot([0 1 1 0 0],[0 0 1 1 0]);
  wires:
  "p{1}"/1 -> mux/1
  mux/1 -> "pd{1,1}"/1
